simulink model "Sistema"  (R2016a)
settings: Solver=VariableStepAuto  StartTime=0.0  StopTime=10.0  RelTol=1e-3
undefined symbols (not defined in the file): Bm, Ea, Jm, Kb, KFi, KPrev, Kt, Kw, La, Ra
settings Model: Creator=Marcelo  LastModifiedBy=Marcelo

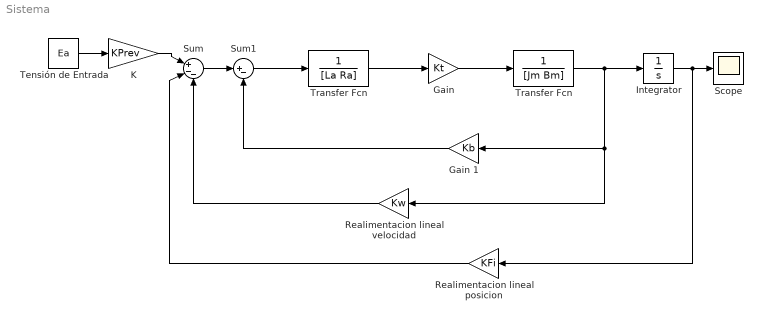
== system Sistema ==
  Gain : Gain  Gain=Kt
  Gain 1 : Gain  Gain=Kb
  Integrator : Integrator
  "K " : Gain  Gain=KPrev
  Realimentacion lineal posicion : Gain  Gain=KFi
  Realimentacion lineal velocidad : Gain  Gain=Kw
  Scope : Scope
  Sum : Sum  Inputs=|+--
  Sum1 : Sum  Inputs=|+-
  Tensión de Entrada : Constant  Value=Ea
  Transfer Fcn : TransferFcn  Denominator=[La Ra]
  "Transfer Fcn " : TransferFcn  Denominator=[Jm Bm]
  wires:
  Sum1/1 -> Transfer Fcn/1
  Gain 1/1 -> Sum1/2
  Transfer Fcn/1 -> Gain/1
  "Transfer Fcn "/1 -> Integrator/1, Gain 1/1, Realimentacion lineal velocidad/1
  Integrator/1 -> Realimentacion lineal posicion/1, Scope/1
  Gain/1 -> "Transfer Fcn "/1
  Sum/1 -> Sum1/1
  Realimentacion lineal velocidad/1 -> Sum/3
  Realimentacion lineal posicion/1 -> Sum/2
  "K "/1 -> Sum/1
  Tensión de Entrada/1 -> "K "/1
